simulink model "Sim1_Supervisor_OA"  (R2021b)
settings: Solver=VariableStepAuto  StartTime=0.0  StopTime=Inf  RelTol=1e-3
StopFcn:
  | %run('AutomoveData.m')
undefined symbols (not defined in the file or in its folder): dt, Sim5_Status, StartSW, Twist
libraries: robotlib x13, sldrtlib x1
settings Model: Creator=shdet  LastModifiedBy=Hibik
settings SolverCC: AlgebraicLoopSolver=TrustRegion
settings DataIOCC: SaveOutput=off  SignalLogging=off  DSMLogging=off  SaveTime=off  ReturnWorkspaceOutputs=off
settings DebuggingCC: PregeneratedLibrarySubsystemCodeDiagnostic=none  SFMachineParentedDataDiag=warning  ArithmeticOperatorsInVariantConditions=warning
settings SFSimCC: SimUseLocalCustomCode=off  CustomCodeUndefinedFunction=UseInterfaceOnly
settings RTWCC: RTWUseLocalCustomCode=off

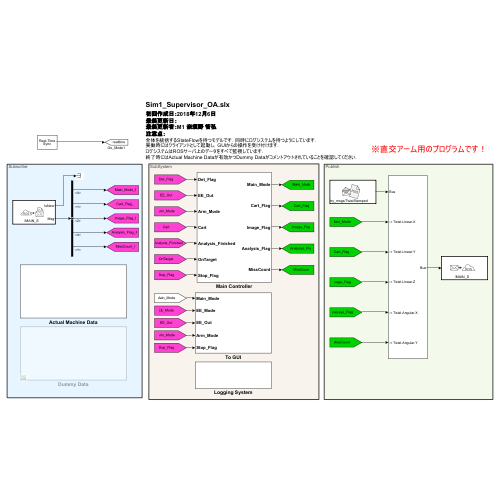
[thumbnail: Simulink's stored preview of the top-level diagram]
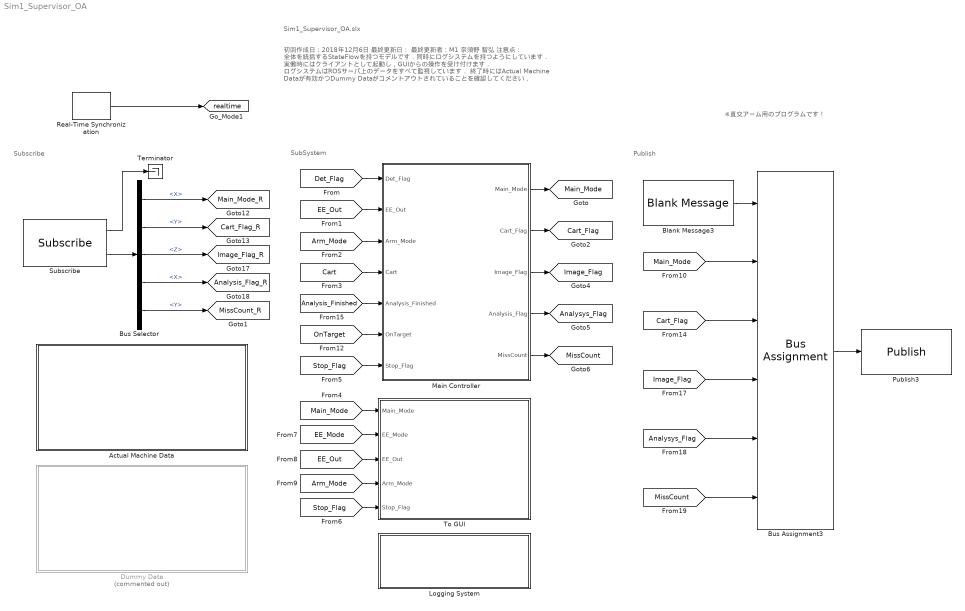
== system Sim1_Supervisor_OA ==
  note: Publish
  note: SubSystem
  note: Sim1_Supervisor_OA.slx
  note: ※直交アーム用のプログラムです！
  note: 初回作成日：2018年12月6日
      | 最終更新日：
      | 最終更新者：M1 奈須野 智弘
      | 注意点：
      | 全体を統括するStateFlowを持つモデルです．同時にログシステムを持つようにしています．
      | 実働時にはクライアントとして起動し，GUIからの操作を受け付けます．
      | ログシステムはROSサーバ上のデータをすべて監視しています．
      | 終了時にはActual Machine Dataが有効かつDummy Dataがコメントアウトされていることを確認してください．
  note: Subscribe
  Actual Machine Data : Subsystem
  Blank Message3 : robotlib/Blank Message  messageClass=Message  entityType=geometry_msgs/TwistStamped  messageType=geometry_msgs/TwistStamped  SampleTime=dt  legacyBusStruct=off
  Bus Assignment3 : BusAssignment  AssignedSignals=Twist.Linear.X,Twist.Linear.Y,Twist.Linear.Z,Twist.Angular.X,Twist.Angular.Y
  Bus Selector : BusSelector  OutputSignals=Twist.Linear.X,Twist.Linear.Y,Twist.Linear.Z,Twist.Angular.X,Twist.Angular.Y
  Dummy Data : Subsystem  Commented=on
  Logging System : Subsystem
  Main Controller : Subsystem
  Publish3 : robotlib/Publish  topicSource=Specify your own  topic=/MAIN_S  messageType=geometry_msgs/TwistStamped  legacyBusStruct=off  messageQueueLength=1
  Real-Time Synchronization : sldrtlib/Real-Time Synchronization  SampleTime=dt  MaxMissedTicks=inf  ShowMissedTicks=on  YieldWhenWaiting=off
  Subscribe : robotlib/Subscribe  topicSource=Specify your own  topic=/MAIN_S  messageType=geometry_msgs/TwistStamped  SampleTime=dt  legacyBusStruct=off  messageQueueLength=1
  Terminator : Terminator
  To GUI : Subsystem
  tag scope: Analysis_Flag_R=global, Analysys_Flag=global, Cart_Flag=global, Cart_Flag_R=global, Image_Flag=global, Image_Flag_R=global, Main_Mode=global, Main_Mode_R=global, MissCount=global, MissCount_R=global, realtime=global
  wires:
  [EE_Out] -> Main Controller/2(EE_Out)
  Bus Selector/3 -> [Image_Flag_R]  "<Z>"
  [Analysis_Finished] -> Main Controller/5(Analysis_Finished)
  [Main_Mode] -> To GUI/1(Main_Mode)
  Real-Time Synchronization/1 -> [realtime]
  Main Controller/4(Analysis_Flag) -> [Analysys_Flag]
  Bus Selector/4 -> [Analysis_Flag_R]  "<X>"
  Main Controller/2(Cart_Flag) -> [Cart_Flag]
  [Det_Flag] -> Main Controller/1(Det_Flag)
  [Arm_Mode] -> To GUI/4(Arm_Mode)
  Main Controller/3(Image_Flag) -> [Image_Flag]
  [Cart] -> Main Controller/4(Cart)
  Main Controller/1(Main_Mode) -> [Main_Mode]
  Bus Selector/2 -> [Cart_Flag_R]  "<Y>"
  [EE_Mode] -> To GUI/2(EE_Mode)
  [Arm_Mode] -> Main Controller/3(Arm_Mode)
  Bus Selector/1 -> [Main_Mode_R]  "<X>"
  Subscribe/1 -> Terminator/1
  Subscribe/2 -> Bus Selector/1
  [EE_Out] -> To GUI/3(EE_Out)
  Bus Selector/5 -> [MissCount_R]  "<Y>"
  Main Controller/5(MissCount) -> [MissCount]
  [OnTarget] -> Main Controller/6(OnTarget)
  Blank Message3/1 -> Bus Assignment3/1
  Bus Assignment3/1 -> Publish3/1
  [Main_Mode] -> Bus Assignment3/2
  [Cart_Flag] -> Bus Assignment3/3
  [Image_Flag] -> Bus Assignment3/4
  [Analysys_Flag] -> Bus Assignment3/5
  [MissCount] -> Bus Assignment3/6
  [Stop_Flag] -> Main Controller/7(Stop_Flag)
  [Stop_Flag] -> To GUI/5(Stop_Flag)

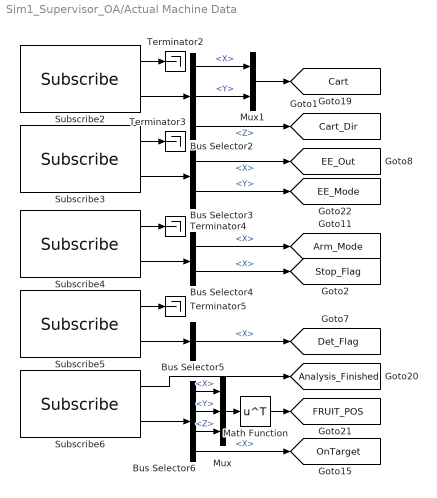
== system Sim1_Supervisor_OA/Actual Machine Data ==
  Bus Selector2 : BusSelector  OutputSignals=Twist.Linear.X,Twist.Linear.Y,Twist.Linear.Z
  Bus Selector3 : BusSelector  OutputSignals=Twist.Linear.X,Twist.Linear.Y
  Bus Selector4 : BusSelector  OutputSignals=Twist.Linear.X,Twist.Angular.X
  Bus Selector5 : BusSelector  OutputSignals=Twist.Linear.X
  Bus Selector6 : BusSelector  OutputSignals=Twist.Linear.X,Twist.Linear.Y,Twist.Linear.Z,Twist.Angular.X
  Math Function : Math  Operator=transpose  SignedPower=on  SaturateOnIntegerOverflow=on
  Mux : Mux  Inputs=3
  Mux1 : Mux  Inputs=2
  Subscribe2 : robotlib/Subscribe  topicSource=Specify your own  topic=/CART_S  messageType=geometry_msgs/TwistStamped  SampleTime=dt  legacyBusStruct=off  messageQueueLength=1
  Subscribe3 : robotlib/Subscribe  topicSource=Specify your own  topic=/EE_S  messageType=geometry_msgs/TwistStamped  SampleTime=dt  legacyBusStruct=off  messageQueueLength=1
  Subscribe4 : robotlib/Subscribe  topicSource=Specify your own  topic=/ARM_S  messageType=geometry_msgs/TwistStamped  SampleTime=dt  legacyBusStruct=off  messageQueueLength=1
  Subscribe5 : robotlib/Subscribe  topicSource=Specify your own  topic=/DET_FLAG_S  messageType=geometry_msgs/TwistStamped  SampleTime=dt  legacyBusStruct=off  messageQueueLength=1
  Subscribe6 : robotlib/Subscribe  topicSource=Specify your own  topic=/FRUIT_POS_S  messageType=geometry_msgs/TwistStamped  SampleTime=dt  legacyBusStruct=off  messageQueueLength=1
  Terminator{2..5} (4 alike) : Terminator
  tag scope: Analysis_Finished=global, Arm_Mode=global, Cart=global, Cart_Dir=global, Det_Flag=global, EE_Mode=global, EE_Out=global, FRUIT_POS=global, OnTarget=global, Stop_Flag=global
  wires:
  Bus Selector4/1 -> [Arm_Mode]  "<X>"
  Subscribe2/1 -> Terminator2/1
  Subscribe3/2 -> Bus Selector3/1
  Subscribe4/1 -> Terminator4/1
  Subscribe2/2 -> Bus Selector2/1
  Bus Selector3/2 -> [EE_Mode]  "<Y>"
  Subscribe3/1 -> Terminator3/1
  Subscribe5/2 -> Bus Selector5/1
  Bus Selector5/1 -> [Det_Flag]  "<X>"
  Bus Selector2/3 -> [Cart_Dir]  "<Z>"
  Bus Selector3/1 -> [EE_Out]  "<X>"
  Subscribe4/2 -> Bus Selector4/1
  Subscribe5/1 -> Terminator5/1
  Mux/1 -> Math Function/1
  Bus Selector6/3 -> Mux/3  "<Z>"
  Subscribe6/2 -> Bus Selector6/1
  Bus Selector6/4 -> [OnTarget]  "<X>"
  Math Function/1 -> [FRUIT_POS]
  Bus Selector6/1 -> Mux/1  "<X>"
  Subscribe6/1 -> [Analysis_Finished]
  Bus Selector6/2 -> Mux/2  "<Y>"
  Bus Selector4/2 -> [Stop_Flag]  "<X>"
  Bus Selector2/1 -> Mux1/1  "<X>"
  Bus Selector2/2 -> Mux1/2  "<Y>"
  Mux1/1 -> [Cart]

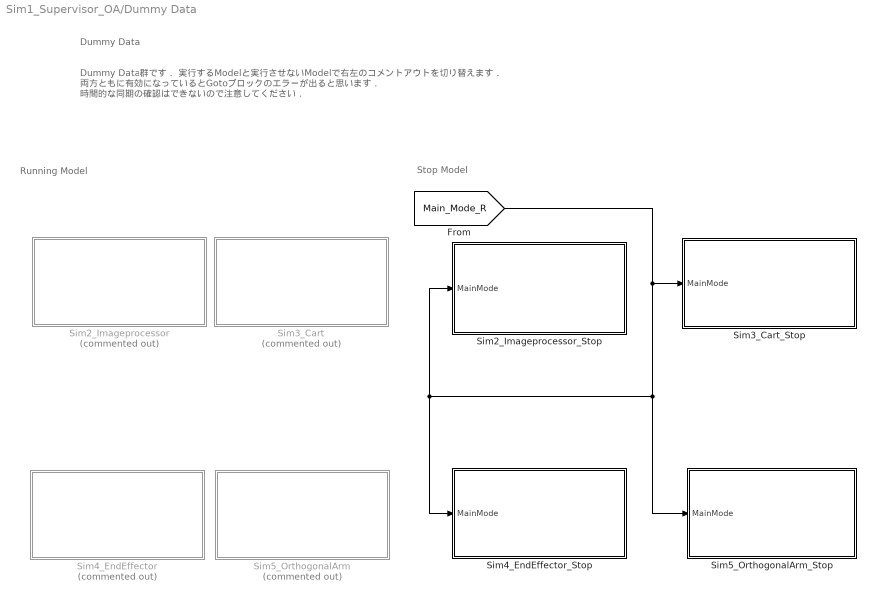
== system Sim1_Supervisor_OA/Dummy Data ==
  note: Dummy Data群です．
      | 実行するModelと実行させないModelで右左のコメントアウトを切り替えます．
      | 両方ともに有効になっているとGotoブロックのエラーが出ると思います．
      | 時間的な同期の確認はできないので注意してください．
  note: Dummy Data
  note: Running Model
  note: Stop Model
  Sim2_Imageprocessor : Subsystem  Commented=on
  Sim2_Imageprocessor_Stop : Subsystem
  Sim3_Cart : Subsystem  Commented=on
  Sim3_Cart_Stop : Subsystem
  Sim4_EndEffector : Subsystem  Commented=on
  Sim4_EndEffector_Stop : Subsystem
  Sim5_OrthogonalArm : Subsystem  Commented=on
  Sim5_OrthogonalArm_Stop : Subsystem
  wires:
  [Main_Mode_R] -> Sim5_OrthogonalArm_Stop/1(MainMode), Sim2_Imageprocessor_Stop/1(MainMode), Sim4_EndEffector_Stop/1(MainMode), Sim3_Cart_Stop/1(MainMode)

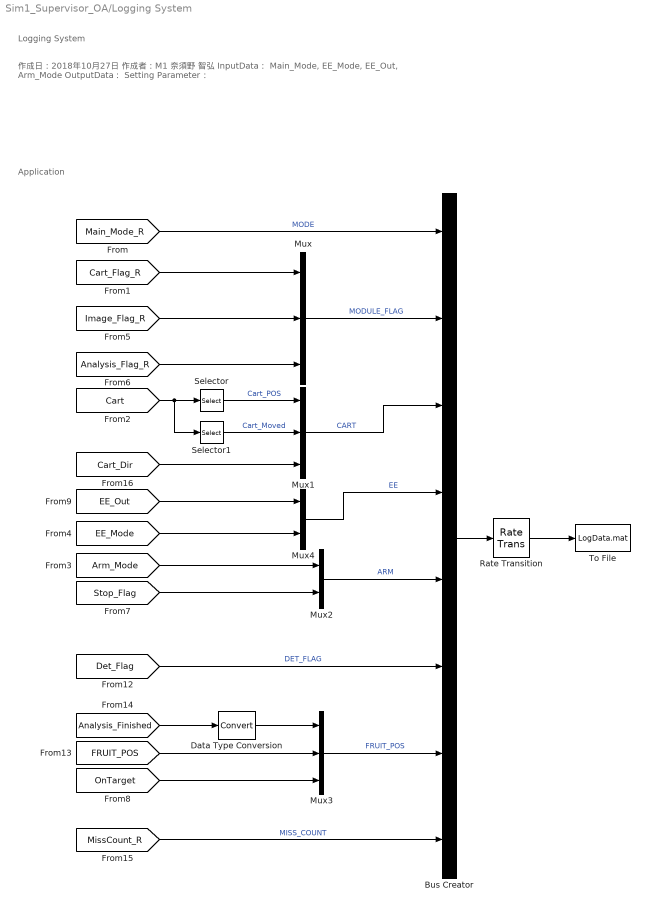
== system Sim1_Supervisor_OA/Logging System ==
  note: Application
  note: 作成日：2018年10月27日
      | 作成者：M1 奈須野 智弘
      |
      | InputData： Main_Mode, EE_Mode, EE_Out, Arm_Mode
      | OutputData：
      | Setting Parameter：
  note: Logging System
  Bus Creator : BusCreator  Inputs=8
  Data Type Conversion : DataTypeConversion
  Mux : Mux  Inputs=3
  Mux1 : Mux  Inputs=3
  Mux2 : Mux  Inputs=2
  Mux3 : Mux  Inputs=3
  Mux4 : Mux  Inputs=2
  Rate Transition : RateTransition
  Selector : Selector  InputPortWidth=2  IndexOptions=Index vector (dialog)  Indices=[1]  OutputSizes=1
  Selector1 : Selector  InputPortWidth=2  IndexOptions=Index vector (dialog)  Indices=[2]  OutputSizes=1
  To File : ToFile  Filename=LogData.mat  MatrixName=LogData  SaveFormat=Timeseries
  wires:
  Bus Creator/1 -> Rate Transition/1
  Rate Transition/1 -> To File/1
  [Main_Mode_R] -> Bus Creator/1  "MODE"
  Mux/1 -> Bus Creator/2  "MODULE_FLAG"
  [Cart_Flag_R] -> Mux/1
  [Image_Flag_R] -> Mux/2
  Selector1/1 -> Mux1/2  "Cart_Moved"
  Mux1/1 -> Bus Creator/3  "CART"
  Mux4/1 -> Bus Creator/4  "EE"
  Mux2/1 -> Bus Creator/5  "ARM"
  [Arm_Mode] -> Mux2/1
  [Stop_Flag] -> Mux2/2
  [Det_Flag] -> Bus Creator/6  "DET_FLAG"
  Mux3/1 -> Bus Creator/7  "FRUIT_POS"
  [Analysis_Finished] -> Data Type Conversion/1
  [FRUIT_POS] -> Mux3/2
  Data Type Conversion/1 -> Mux3/1
  [Cart_Dir] -> Mux1/3
  [EE_Mode] -> Mux4/2
  [EE_Out] -> Mux4/1
  [MissCount_R] -> Bus Creator/8  "MISS_COUNT"
  [Analysis_Flag_R] -> Mux/3
  [Cart] -> Selector1/1, Selector/1
  Selector/1 -> Mux1/1  "Cart_POS"
  [OnTarget] -> Mux3/3

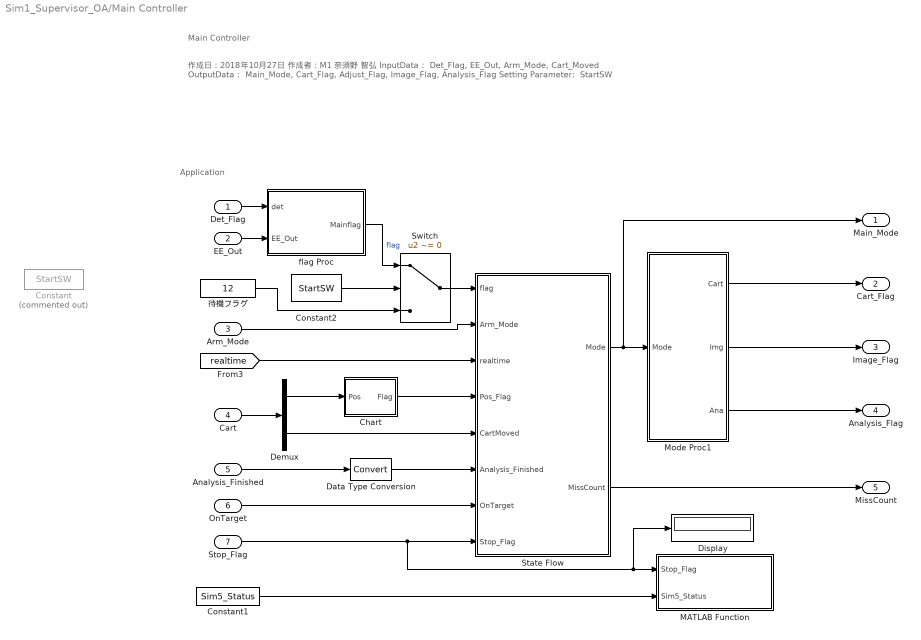
== system Sim1_Supervisor_OA/Main Controller ==
  note: Application
  note: 作成日：2018年10月27日
      | 作成者：M1 奈須野 智弘
      |
      | InputData： Det_Flag, EE_Out, Arm_Mode, Cart_Moved
      | OutputData： Main_Mode, Cart_Flag, Adjust_Flag, Image_Flag, Analysis_Flag
      | Setting Parameter： StartSW
  note: Main Controller
  Det_Flag : Inport
  EE_Out : Inport  Port=2
  Arm_Mode : Inport  Port=3
  Cart : Inport  Port=4
  Analysis_Finished : Inport  Port=5
  OnTarget : Inport  Port=6
  Stop_Flag : Inport  Port=7
  Chart : Stateflow chart  TreatAsAtomicUnit=on
  Constant : Constant  Commented=on  Value=StartSW  SampleTime=Inf
  Constant1 : Constant  Value=Sim5_Status  SampleTime=dt
  Constant2 : Constant  Value=StartSW
  Data Type Conversion : DataTypeConversion
  Demux : Demux  Outputs=2
  Display : Display
  MATLAB Function : MATLAB Function  TreatAsAtomicUnit=on
  Mode Proc1 : MATLAB Function  TreatAsAtomicUnit=on
  State Flow : Stateflow chart  TreatAsAtomicUnit=on
  Switch : Switch  Criteria=u2 ~= 0
  flag Proc : MATLAB Function  TreatAsAtomicUnit=on
  待機フラグ : Constant  Value=12
  Main_Mode : Outport  VectorParamsAs1DForOutWhenUnconnected=off
  Cart_Flag : Outport  Port=2  VectorParamsAs1DForOutWhenUnconnected=off
  Image_Flag : Outport  Port=3  VectorParamsAs1DForOutWhenUnconnected=off
  Analysis_Flag : Outport  Port=4  VectorParamsAs1DForOutWhenUnconnected=off
  MissCount : Outport  Port=5  VectorParamsAs1DForOutWhenUnconnected=off
  wires:
  [realtime] -> State Flow/3(realtime)
  Cart/1 -> Demux/1
  EE_Out/1 -> flag Proc/2(EE_Out)
  Switch/1 -> State Flow/1(flag)
  flag Proc/1(Mainflag) -> Switch/1  "flag"
  Arm_Mode/1 -> State Flow/2(Arm_Mode)
  待機フラグ/1 -> Switch/3
  Det_Flag/1 -> flag Proc/1(det)
  Mode Proc1/1(Cart) -> Cart_Flag/1
  Mode Proc1/2(Img) -> Image_Flag/1
  Mode Proc1/3(Ana) -> Analysis_Flag/1
  Analysis_Finished/1 -> Data Type Conversion/1
  Data Type Conversion/1 -> State Flow/6(Analysis_Finished)
  OnTarget/1 -> State Flow/7(OnTarget)
  State Flow/2(MissCount) -> MissCount/1
  Chart/1(Flag) -> State Flow/4(Pos_Flag)
  Demux/2 -> State Flow/5(CartMoved)
  Demux/1 -> Chart/1(Pos)
  Stop_Flag/1 -> Display/1, MATLAB Function/1(Stop_Flag), State Flow/8(Stop_Flag)
  State Flow/1(Mode) -> Mode Proc1/1(Mode), Main_Mode/1
  Constant1/1 -> MATLAB Function/2(Sim5_Status)
  Constant2/1 -> Switch/2

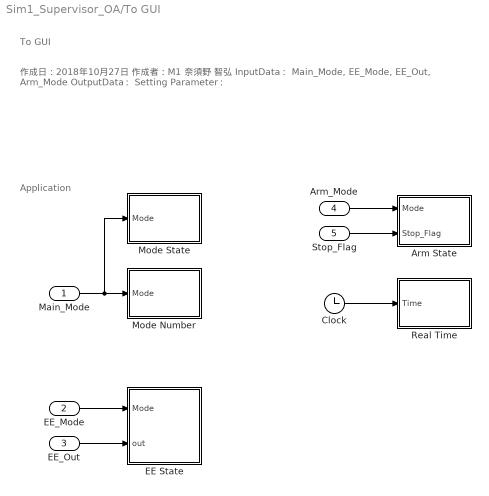
== system Sim1_Supervisor_OA/To GUI ==
  note: Application
  note: 作成日：2018年10月27日
      | 作成者：M1 奈須野 智弘
      |
      | InputData： Main_Mode, EE_Mode, EE_Out, Arm_Mode
      | OutputData：
      | Setting Parameter：
  note: To GUI
  Main_Mode : Inport
  EE_Mode : Inport  Port=2
  EE_Out : Inport  Port=3
  Arm_Mode : Inport  Port=4
  Stop_Flag : Inport  Port=5
  Arm State : MATLAB Function  TreatAsAtomicUnit=on
  Clock : Clock
  EE State : MATLAB Function  TreatAsAtomicUnit=on
  Mode Number : MATLAB Function  TreatAsAtomicUnit=on
  Mode State : MATLAB Function  TreatAsAtomicUnit=on
  Real Time : MATLAB Function  TreatAsAtomicUnit=on
  wires:
  Main_Mode/1 -> Mode State/1(Mode), Mode Number/1(Mode)
  EE_Mode/1 -> EE State/1(Mode)
  Arm_Mode/1 -> Arm State/1(Mode)
  EE_Out/1 -> EE State/2(out)
  Clock/1 -> Real Time/1(Time)
  Stop_Flag/1 -> Arm State/2(Stop_Flag)

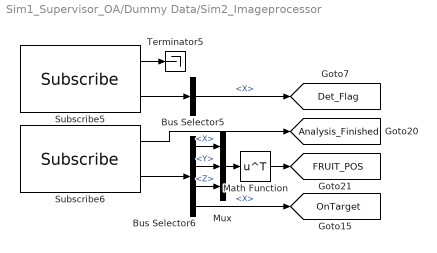
== system Sim1_Supervisor_OA/Dummy Data/Sim2_Imageprocessor ==
  Bus Selector5 : BusSelector  OutputSignals=Twist.Linear.X
  Bus Selector6 : BusSelector  OutputSignals=Twist.Linear.X,Twist.Linear.Y,Twist.Linear.Z,Twist.Angular.X
  Math Function : Math  Operator=transpose  SignedPower=on  SaturateOnIntegerOverflow=on
  Mux : Mux  Inputs=3
  Subscribe5 : robotlib/Subscribe  topicSource=Specify your own  topic=/DET_FLAG_S  messageType=geometry_msgs/TwistStamped  SampleTime=dt  legacyBusStruct=off  messageQueueLength=1
  Subscribe6 : robotlib/Subscribe  topicSource=Specify your own  topic=/FRUIT_POS_S  messageType=geometry_msgs/TwistStamped  SampleTime=dt  legacyBusStruct=off  messageQueueLength=1
  Terminator5 : Terminator
  tag scope: Analysis_Finished=global, Det_Flag=global, FRUIT_POS=global, OnTarget=global
  wires:
  Subscribe5/2 -> Bus Selector5/1
  Subscribe5/1 -> Terminator5/1
  Bus Selector5/1 -> [Det_Flag]  "<X>"
  Mux/1 -> Math Function/1
  Bus Selector6/3 -> Mux/3  "<Z>"
  Subscribe6/2 -> Bus Selector6/1
  Bus Selector6/4 -> [OnTarget]  "<X>"
  Math Function/1 -> [FRUIT_POS]
  Bus Selector6/1 -> Mux/1  "<X>"
  Subscribe6/1 -> [Analysis_Finished]
  Bus Selector6/2 -> Mux/2  "<Y>"

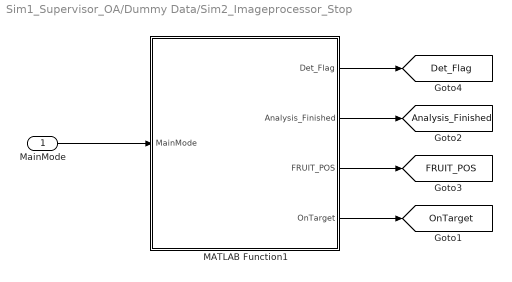
== system Sim1_Supervisor_OA/Dummy Data/Sim2_Imageprocessor_Stop ==
  MainMode : Inport
  MATLAB Function1 : MATLAB Function  TreatAsAtomicUnit=on
  tag scope: Analysis_Finished=global, Det_Flag=global, FRUIT_POS=global, OnTarget=global
  wires:
  MATLAB Function1/3(FRUIT_POS) -> [FRUIT_POS]
  MATLAB Function1/2(Analysis_Finished) -> [Analysis_Finished]
  MATLAB Function1/4(OnTarget) -> [OnTarget]
  MATLAB Function1/1(Det_Flag) -> [Det_Flag]
  MainMode/1 -> MATLAB Function1/1(MainMode)

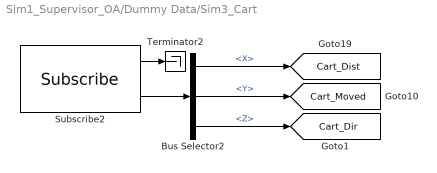
== system Sim1_Supervisor_OA/Dummy Data/Sim3_Cart ==
  Bus Selector2 : BusSelector  OutputSignals=Twist.Linear.X,Twist.Linear.Y,Twist.Linear.Z
  Subscribe2 : robotlib/Subscribe  topicSource=Specify your own  topic=/CART_S  messageType=geometry_msgs/TwistStamped  SampleTime=dt  legacyBusStruct=off  messageQueueLength=1
  Terminator2 : Terminator
  tag scope: Cart_Dir=global, Cart_Dist=global, Cart_Moved=global
  wires:
  Bus Selector2/1 -> [Cart_Dist]  "<X>"
  Bus Selector2/2 -> [Cart_Moved]  "<Y>"
  Subscribe2/2 -> Bus Selector2/1
  Bus Selector2/3 -> [Cart_Dir]  "<Z>"
  Subscribe2/1 -> Terminator2/1

== system Sim1_Supervisor_OA/Dummy Data/Sim3_Cart_Stop ==
  MainMode : Inport
  MATLAB Function : MATLAB Function  TreatAsAtomicUnit=on
  tag scope: Cart=global
  wires:
  MainMode/1 -> MATLAB Function/1(MainMode)
  MATLAB Function/1(Cart) -> [Cart]

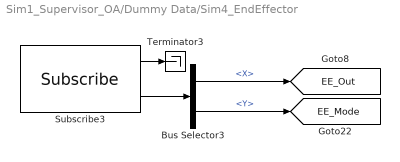
== system Sim1_Supervisor_OA/Dummy Data/Sim4_EndEffector ==
  Bus Selector3 : BusSelector  OutputSignals=Twist.Linear.X,Twist.Linear.Y
  Subscribe3 : robotlib/Subscribe  topicSource=Specify your own  topic=/EE_S  messageType=geometry_msgs/TwistStamped  SampleTime=dt  legacyBusStruct=off  messageQueueLength=1
  Terminator3 : Terminator
  tag scope: EE_Mode=global, EE_Out=global
  wires:
  Subscribe3/1 -> Terminator3/1
  Bus Selector3/1 -> [EE_Out]  "<X>"
  Subscribe3/2 -> Bus Selector3/1
  Bus Selector3/2 -> [EE_Mode]  "<Y>"

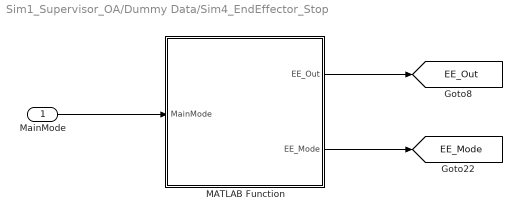
== system Sim1_Supervisor_OA/Dummy Data/Sim4_EndEffector_Stop ==
  MainMode : Inport
  MATLAB Function : MATLAB Function  TreatAsAtomicUnit=on
  tag scope: EE_Mode=global, EE_Out=global
  wires:
  MainMode/1 -> MATLAB Function/1(MainMode)
  MATLAB Function/1(EE_Out) -> [EE_Out]
  MATLAB Function/2(EE_Mode) -> [EE_Mode]

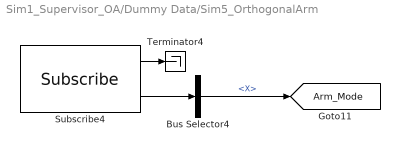
== system Sim1_Supervisor_OA/Dummy Data/Sim5_OrthogonalArm ==
  Bus Selector4 : BusSelector  OutputSignals=Twist.Linear.X
  Subscribe4 : robotlib/Subscribe  topicSource=Specify your own  topic=/ARM_S  messageType=geometry_msgs/TwistStamped  SampleTime=dt  legacyBusStruct=off  messageQueueLength=1
  Terminator4 : Terminator
  tag scope: Arm_Mode=global
  wires:
  Subscribe4/2 -> Bus Selector4/1
  Subscribe4/1 -> Terminator4/1
  Bus Selector4/1 -> [Arm_Mode]  "<X>"

== system Sim1_Supervisor_OA/Dummy Data/Sim5_OrthogonalArm_Stop ==
  MainMode : Inport
  MATLAB Function : MATLAB Function  TreatAsAtomicUnit=on
  tag scope: Arm_Mode=global
  wires:
  MainMode/1 -> MATLAB Function/1(MainMode)
  MATLAB Function/1(Arm_Mode) -> [Arm_Mode]

== stateflow chart Sim1_Supervisor_OA/Main Controller/State Flow ==
  state CheckRealtime/
    entry:Mode=-100;
  state Mode10/
    entry:Mode=10;
    % 動作準備モード
    state Mode11/
      entry:Mode=11;
      % Armキャリブレーション_Arm
    state Mode12/
      entry:Mode=12;
      MissCount = 0;
      % 待機
    (default) -> Mode11
    Mode11 -> Mode12 : [Arm_Mode == 100]
    Mode12 -> Mode12 [order 2] : [flag == 12]
  state Mode40/
    entry:Mode=40;
    % 収穫モード
    state Mode41/
      entry:Mode=41;
      % Arm(yz)移動_Arm
    state Mode42/
      entry:Mode=42;
      % Arm(x)移動・吸引_Arm, EE
    state wait40/
      entry:Mode=-40;
    state Mode43/
      entry:Mode=43;
      % EE閉_EE
    state Mode47/
      entry:
      Mode=47;
      combo = 0;
      % 収穫失敗
      % 吸引なし
    state Mode45/
      entry:Mode=45;
      % 把持_EE
    (default) -> Mode41
    Mode41 -> Mode42 : after(1,sec)
        | [Arm_Mode == 3]
    Mode42 -> wait40 : after(1,sec)
        | [Arm_Mode == 10]
    wait40 -> Mode43 [order 1] : [flag == 43]
        | % flag==43 : 光センサ反応
    wait40 -> Mode47 [order 2] : after(3.5,sec)
    Mode43 -> Mode45 : % 上EESW反応
        | after(7.0,sec)
        | [flag == 44]
    Mode45 -> Mode47 [order 2] : % 把持失敗
        | after(2,sec)
        | [flag == 46]
  state Mode20/
    entry:Mode=20;
    % 探索モード
    state Mode21/
      entry:Mode=21;
      % 微小移動_Cart
    state Mode22/
      entry:Mode=22;
      % トマト探索_Cart, Img
    (default) -> Mode21
    Mode21 -> Mode22 : after(4.0,sec)[Pos_Flag > 0]
  state Mode50/
    entry:Mode=50;
    % 完了モード
    state Mode51/
      entry:Mode=51;
      % Arm収穫BOXへ移動
    state wait50/
      entry:Mode=-50;
    state Mode52/
      entry:
      Mode=52;
      combo=0;
      MissCount = MissCount + 1;
    (default) -> Mode51
    Mode51 -> wait50 : after(1,sec)
        | [Arm_Mode == 22]
    wait50 -> Mode52 [order 2]
  state Mode60/
    entry:Mode=60;
    % 果実誘導モード
    state Mode61/
      entry:Mode = 61;
      %EE開_EE
    state Mode62/
      entry:
      Mode=62;
      combo = combo + 1;
      % Arm初期位置へ移動
    (default) -> Mode61
    Mode61 -> Mode62 : [flag == 62 || flag == 70]
        | %flag62 トマトが落下した
        | %flag70 下EESW反応
  state Mode30/
    entry:Mode=30;
    % 解析・微調整モード
    state Mode31/
      entry:Mode=31;
      %カートの停止待ち_Cart
    note: CartMoved =- 1
    state Mode32/
      entry:Mode=32;
      %画像取得_Img
    state Mode33/
      entry:Mode=33;
      % 目標トマト果実位置の検出_Ana
    (default) -> Mode31
    Mode31 -> Mode32 : [CartMoved == 1]
    Mode32 -> Mode33 [order 1] : after(0.5,sec)[flag==30]
  state ResetMissCount/
    entry:
    MissCount = 0;
  note: アームx軸を初期位置まで移動
  state Mode70/
    entry:
    Mode=70;
    % 終了モード
  (default) -> CheckRealtime
  Mode20 -> CheckRealtime : [realtime >10000]
  CheckRealtime -> CheckRealtime [order 2]
  CheckRealtime -> Mode10 [order 1] : [realtime < 10000]
      | {
      | MissCount = 0;
      | combo = 0;
      | }
  Mode70 -> Mode12 [order 2] : after(1,sec)
      | [flag == 12&&Arm_Mode==100]
  Mode12 -> Mode20 [order 1] : [flag ~= 12]
  Mode40 -> (junction 334) : [Stop_Flag == 1]
  Mode33 -> Mode40 [order 1] : after(1,sec)
      | [Analysis_Finished == 1 && OnTarget == 1]
  ResetMissCount -> Mode20
  Mode47 -> (junction 323) : after(1,sec)[flag == 46 || Arm_Mode == 22]
  Mode45 -> Mode50 [order 1] : % 把持成功
      | after(2,sec)
      | [flag == 50]
  Mode22 -> Mode30 : [flag == 30]
  Mode70 -> Mode32 [order 1] : after(0.5,sec)
      | [(combo>0 || (MissCount>0&&MissCount<3)) && Arm_Mode == 100]
  Mode32 -> ResetMissCount [order 2] : after(2.5,sec)[flag~=30]
  wait50 -> Mode60 [order 1] : [flag == 50]
      | % 光センサが反応・EE内に果実が存在
  Mode33 -> ResetMissCount [order 2] : after(2.0,sec)
      | [Analysis_Finished == 1 && OnTarget == 0]
  Mode70 -> ResetMissCount [order 3] : after(1.5,sec)
      | [Arm_Mode==100]
  Mode60 -> (junction 334) : [Stop_Flag == 1]
  (junction 334) -> (junction 339)
  Mode62 -> Mode70 : after(1,sec)
      | [Arm_Mode == 33 && flag == 70]
  (junction 323) -> Mode52
  Mode50 -> (junction 339) : [Stop_Flag == 1]
  Mode52 -> Mode70 : after(1,sec)[Arm_Mode == 33]
  (junction 339) -> Mode70
  data: Mode output; flag input; Arm_Mode input; realtime input; Pos_Flag input; CartMoved input; Analysis_Finished input; OnTarget input; MissCount output; combo local; Stop_Flag input

== stateflow chart Sim1_Supervisor_OA/Main Controller/Chart ==
  state Wait1/
    entry:
    Flag = 0;
  state Wait/
    entry:
    Flag = 1;
  (default) -> Wait1
  Wait1 -> Wait : [Pos > -1.0]
  data: Pos input; Flag output

== matlab function Sim1_Supervisor_OA/Dummy Data/Sim3_Cart_Stop/MATLAB Function ==
  data: MainMode input; Cart output
function Cart  = fcn(MainMode)

Cart = [0, 0];

if MainMode > 30
    Cart(2) = 1;
end

Cart(1) = randi(100);

== matlab function Sim1_Supervisor_OA/Dummy Data/Sim4_EndEffector_Stop/MATLAB Function ==
  data: MainMode input; EE_Out output; EE_Mode output
function [EE_Out, EE_Mode] = fcn(MainMode)

EE_Out = 0;
EE_Mode = 0;

if MainMode == -40
    EE_Out = 5;
elseif MainMode == 43
    EE_Out = 6;
elseif MainMode == 45 || MainMode == -50
    EE_Out = 4;
elseif MainMode == 61
    EE_Out = 8;
elseif MainMode == 62
    EE_Out = 7;
end

if MainMode == 42
    EE_Mode = 1;
elseif MainMode == 43
    EE_Mode = 2;
elseif MainMode == 45
    EE_Mode = 4;
elseif MainMode == 61
    EE_Mode = 3;
end

== matlab function Sim1_Supervisor_OA/Main Controller/Mode Proc1 ==
  data: Mode input; Cart output; Img output; Ana output
function [Cart, Img, Ana] = fcn(Mode)

Cart = 0;
Img = 0;
Ana = 0;

% Cart
if Mode==21
    % 微小移動_Cart
    Cart = 1;
    
% Cart, Img
elseif Mode==22
    % トマト探索_Cart, Img
    Cart = 1;
    Img = 1;

% Ana
elseif Mode==32 || Mode==35
    % 解析モード
    % 解析に用いる画像の取得_Img
    Img = 1;

elseif Mode==33 || Mode==36
    % 目標トマト果実位置の検出_Ana
    Ana = 1;
  
% No
else
    Cart = 0;
    Img = 0;
    Ana = 0;
end

== matlab function Sim1_Supervisor_OA/Dummy Data/Sim5_OrthogonalArm_Stop/MATLAB Function ==
  data: MainMode input; Arm_Mode output; Stop_Flag output
function  [Arm_Mode, Stop_Flag] = fcn(MainMode)

Arm_Mode = 0;
Stop_Flag = 0;

if MainMode == 41
    Arm_Mode = 41;
elseif MainMode == 42
    Arm_Mode = 42;
elseif MainMode == 46
    Arm_Mode = 44;
elseif MainMode == 62
    Arm_Mode = 61;
elseif MainMode == 51 || MainMode == 65
    Arm_Mode = 99;
else
    Arm_Mode = 40;
end

== matlab function Sim1_Supervisor_OA/Dummy Data/Sim2_Imageprocessor_Stop/MATLAB Function1 ==
  data: MainMode input; Det_Flag output; Analysis_Finished output; FRUIT_POS output; OnTarget output
function [Det_Flag, Analysis_Finished, FRUIT_POS, OnTarget] = fcn(MainMode)

Det_Flag = 0;
Analysis_Finished = 0;
FRUIT_POS = [150,0,280];
OnTarget = 0;

if MainMode == 22 || MainMode == 32 || MainMode == 35
    Det_Flag = 1;
end

if MainMode == 33 || MainMode == 36
    Analysis_Finished = 1;
end

if MainMode == 33 || MainMode == 36
    OnTarget = 1;
end

== matlab function Sim1_Supervisor_OA/Main Controller/flag Proc ==
  data: det input; Mainflag output; EE_Out input
function Mainflag = fcn(det, EE_Out)

% トマト果実検出
if det== 1
    Mainflag = 30;
% 把持中(EE_Mode4にて、光センサが反応・EE内に果実が存在)
elseif EE_Out == 4
    Mainflag = 50;
% センサ反応
elseif EE_Out == 5
    Mainflag = 43;
% 上SW反応(EEが閉じた状態)
elseif EE_Out == 6
    Mainflag = 44;
% 下SW反応(EEが開いた状態)
elseif EE_Out == 7
    Mainflag = 70;
% 吸引終了，トマト落下確認（    
elseif EE_Out == 8
    Mainflag = 62;
% 把持失敗(EE_Mode4にて、光センサが反応せず)
elseif EE_Out == 0
    Mainflag = 46;
else
    Mainflag = -1;
end

== matlab function Sim1_Supervisor_OA/Main Controller/MATLAB Function ==
  data: Stop_Flag input; Sim5_Status input
function fcn(Stop_Flag, Sim5_Status)

coder.extrinsic('set_param');

if Sim5_Status == 0 && Stop_Flag == 1
    set_param('Sim5_OrthogonalArm_XY_OA','SimulationCommand','Stop');
elseif Sim5_Status == 1
    set_param('Sim5_OrthogonalArm_XY_OA','SimulationCommand','Start');
end

== matlab function Sim1_Supervisor_OA/To GUI/Mode Number ==
  data: Mode input

function fcn(Mode)

% GUIへ値の送信
% edit1 -> Mode Nymber
coder.extrinsic('num2str');
set(findobj('tag','ModeNum'),'string',num2str(Mode));

== matlab function Sim1_Supervisor_OA/To GUI/Mode State ==
  data: Mode input

function fcn(Mode)

% GUIへ値の送信
% 10~：動作準備モード
% 20~：探索モード
% 30~：解析モード
% 40~：収穫モード
% 50~：完了モード
% 60~：果実誘導モード
% 70~：終了モード

% 10~：動作準備モード
if Mode == 10
    set(findobj('tag','State'),'string','Preparation Mode');
elseif Mode == 11
    set(findobj('tag','State'),'string','Calibration');
elseif Mode == 12
    set(findobj('tag','State'),'string','Wait');
% 20~：探索モード
elseif Mode == 20
    set(findobj('tag','State'),'string','Search Mode');
elseif Mode == 21
    set(findobj('tag','State'),'string','Movement_Cart(y)');
elseif Mode == 22
    set(findobj('tag','State'),'string','Search of tomato');
% 30~：解析モード
elseif Mode == 30
    set(findobj('tag','State'),'string','Analysis Mode');
elseif Mode == 31
    set(findobj('tag','State'),'string','Wait for Cart');
elseif Mode == 32
    set(findobj('tag','State'),'string','Get the Image');
elseif Mode == 33
    set(findobj('tag','State'),'string','Detection of target tomato');
% 40~：収穫モード
elseif Mode == 40
    set(findobj('tag','State'),'string','Harvesting Mode'); 
elseif Mode == 41
    set(findobj('tag','State'),'string','Movement_Arm(yz)'); 
elseif Mode == 42
    set(findobj('tag','State'),'string','Movement_Arm(x)'); 
elseif Mode == 43
    set(findobj('tag','State'),'string','Close EE'); 
elseif Mode == 45
    set(findobj('tag','State'),'string','Movement_Arm(yz)');
elseif Mode == 46
    set(findobj('tag','State'),'string','Additional move');  
elseif Mode == 47
    set(findobj('tag','State'),'string','Failed');  
elseif Mode == -40
    set(findobj('tag','State'),'string','Wait for Getting Fruit');
% 50~：完了モード 
elseif Mode == 50
    set(findobj('tag','State'),'string','Compreat');
elseif Mode == 51
    set(findobj('tag','State'),'string','Movement_Arm(BOX)');
elseif Mode == 52
    set(findobj('tag','State'),'string','Add MissCount');
elseif Mode == -50
    set(findobj('tag','State'),'string','Wait');
% 60~：果実誘導モード 
elseif Mode == 60
    set(findobj('tag','State'),'string','Tomato guidance');
elseif Mode == 61
    set(findobj('tag','State'),'string','Open EE');    
elseif Mode == 62
    set(findobj('tag','State'),'string','Movement_Arm(Initial)');
% 70~：終了モード
elseif Mode == 70
    set(findobj('tag','State'),'string','Finish');   
else
    set(findobj('tag','State'),'string','NaN');
end

== matlab function Sim1_Supervisor_OA/To GUI/EE State ==
  data: Mode input; out input

function fcn(Mode,out)

% GUIへ値の送信


% 0：待機モード
if Mode == 0
    if out == 0
        set(findobj('tag','EEState'),'string','Wait(EDF Off)');
    else
        set(findobj('tag','EEState'),'string','NaN');
    end
    
% 1：吸引モード（1：センサ未反応　5：センサ反応）
elseif Mode == 1
    if out == 1
        set(findobj('tag','EEState'),'string','Suction(EDF On)');
    elseif out == 5
        set(findobj('tag','EEState'),'string','Sensor On(EDF On)');
    else
        set(findobj('tag','EEState'),'string','NaN');
    end
    
% 2：切断モード（閉）
elseif Mode == 2
    if out == 2
        set(findobj('tag','EEState'),'string','EE Closing(EDF On)');
    elseif out == 6
        set(findobj('tag','EEState'),'string','EE Closed(EDF On)');
    else
        set(findobj('tag','EEState'),'string','NaN');
    end
    
% 3：切断モード（開）   
elseif Mode == 3
    if out == 3
        set(findobj('tag','EEState'),'string','EE Opening(EDF Off)');
    elseif out == 7
        set(findobj('tag','EEState'),'string','EE Opened(EDF Off)');
    elseif out == 8
        set(findobj('tag','EEState'),'string','EE Opened(Fruit Drop)');
    else
        set(findobj('tag','EEState'),'string','NaN');
    end
    
% 4：把持
elseif Mode == 4
    if out == 4
        set(findobj('tag','EEState'),'string','Catch the Fruit');
    elseif out == 0
        set(findobj('tag','EEState'),'string','Can not Catch');
    else
        set(findobj('tag','EEState'),'string','NaN');
    end
else
    set(findobj('tag','EEState'),'string','NaN');
end

== matlab function Sim1_Supervisor_OA/To GUI/Arm State ==
  data: Mode input; Stop_Flag input

function fcn(Mode, Stop_Flag)

% GUIへ値の送信

if Stop_Flag == 1
    set(findobj('tag','ArmState'),'string','Connect Error');
else    
    %100：待機
    if Mode == 100
        set(findobj('tag','ArmState'),'string','Wait');

    %1：Arm(y)ターゲットへ移動
    elseif Mode == 1
        set(findobj('tag','ArmState'),'string','Move (y) to Target'); 

    %2：Arm(z)ターゲットへ移動
    elseif Mode == 2
        set(findobj('tag','ArmState'),'string','Move (z) to Target');

    %3：Arm(z)ターゲットへ移動完了
    elseif Mode == 3
        set(findobj('tag','ArmState'),'string','Finished (z)');

    %4：Arm(x)ターゲットへ移動
    elseif Mode == 4
        set(findobj('tag','ArmState'),'string','Move (x) to Target');

    %10：果実座標へ移動完了 
    elseif Mode == 10
        set(findobj('tag','ArmState'),'string','Finished (x)');

    %11：Arm(x)BOXへ移動
    elseif Mode == 11
        set(findobj('tag','ArmState'),'string','Move (x) to BOX');

    %12：Arm(y)BOXへ移動
    elseif Mode == 12
        set(findobj('tag','ArmState'),'string','Move (y) to BOX');

    %13：Arm(z)BOXへ移動
    elseif Mode == 13
        set(findobj('tag','ArmState'),'string','Move (z) to BOX');

    %20：収穫箱への移動完了
    elseif Mode == 20
        set(findobj('tag','ArmState'),'string','Finished moving to BOX');

    %：Arm初期位置帰還
    elseif Mode == -1
        set(findobj('tag','ArmState'),'string','Return Init. Pos.(Error)');

    elseif Mode == 21
        set(findobj('tag','ArmState'),'string','Return Init. (x)');

    elseif Mode == 22
        set(findobj('tag','ArmState'),'string','Return Init. (y)');

    elseif Mode == 23
        set(findobj('tag','ArmState'),'string','Return Init. (z)');

    %30：Arm初期位置移動完了
    elseif Mode == 30
        set(findobj('tag','ArmState'),'string','Finished returning Init. Pos');

    %：Arm初期位置帰還(未終了)    
    elseif Mode == 41
        set(findobj('tag','ArmState'),'string','Return Init. (x) Error');

    elseif Mode == 42
        set(findobj('tag','ArmState'),'string','Return Init. (y) Error');

    elseif Mode == 43
        set(findobj('tag','ArmState'),'string','Return Init. (z) Error');

    else
        set(findobj('tag','ArmState'),'string','NaN');
    end
end

== matlab function Sim1_Supervisor_OA/To GUI/Real Time ==
  data: Time input

function fcn(Time)

% GUIへ値の送信

coder.extrinsic('num2str');
set(findobj('tag','RealTime'),'string',num2str(Time));
